simulink model "quad_tank_plant_full_sim"  (R2026a)
settings: Solver=VariableStepAuto  StopTime=120
values from neighbouring files (symbols this model uses):
  a1 = (a11 + a12)/2    [areas.m]    (also in parametros.m = 0.0006136)
  A2 = 0.159    [parametros.m]
  a2 = mean([a21 a22],2)    [areas.m]    (also in parametros.m = 0.00054678)
  A3 = 0.159    [parametros.m]
  a3 = mean([a31 a32],2)    [areas.m]    (also in parametros.m = 0.00035752; prbs_calc_L3.m = 0.00035752; ti_calc.m = 0.00035752)
  A4 = 0.159    [parametros.m]
  a4 = mean([a41 a42],2)    [areas.m]    (also in parametros.m = 0.0004182; ti_calc.m = 0.0004182)
  g = 9.81    [areas.m]    (also in parametros.m; prbs_calc_L3.m; ti_calc.m)
  gamma1 = 0.455    [areas.m]    (also in parametros.m)
  gamma2 = 0.4195    [areas.m]    (also in parametros.m)
  h_max = 0.6    [areas.m]    (also in parametros.m)
  k1 = q_max    (= 0.0017)    [areas.m]    (also in parametros.m)
  k2 = q_max    (= 0.0017)    [areas.m]    (also in parametros.m)
  q_max = 0.0017    [areas.m]    (also in parametros.m)
undefined symbols (not defined in the file or in its folder): A1
libraries: slpidlib x8, simulink x2
settings Model: Creator=agusc  LastModifiedBy=agusc

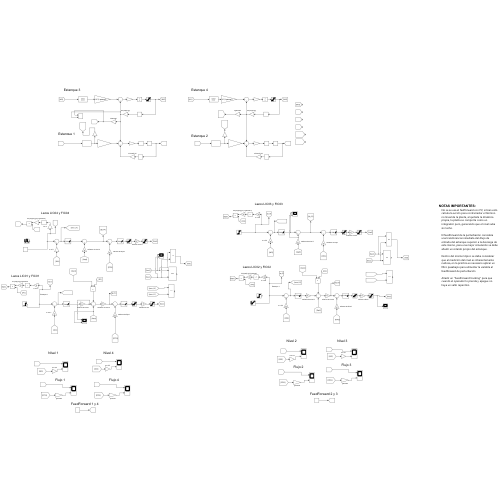
[thumbnail: Simulink's stored preview of the top-level diagram]
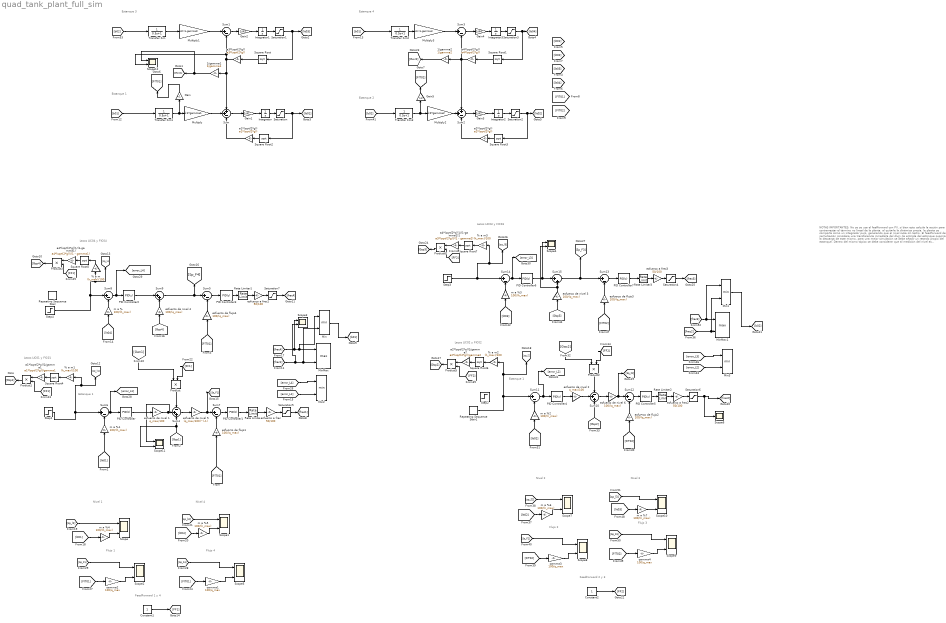
== system quad_tank_plant_full_sim ==
  note: NOTAS IMPORTANTES:
      | No se se usa el feefforward con PV, si bien esto calcula la acción para contrarrestar el término no lineal de la planta, al quitarle la dinámica propia, la planta se comporta como un integrador puro, generando que el nivel suba sin techo.
      |
      | El feedforward de la perturbación considera una transferencia inmediata del dlujo de entrada del estanque superior a la descarga de este mismo, para una mejor simulación se debe añadir un retardo propio del estanque.
      |
      | Dentro del mismo tópico se debe considerar que al medición del nivel es inherentemente ruidosa, en la práctica es necesario aplicar un filtro pasabajos para alimentar la variable al feedforward de perturbación
      |
      | Añadir un "Feedforward tracking" para que cuando el operador lo prenda y apague no haya un salto repentino
  note: Nivel 1
  note: Lazos LIC01 y FIC01
  note: Estanque 2
  note: Estanque 4
  note: Estanque 3
  note: Estanque 1
  note: Estanque 1
  note: Flujo 1
  note: Nivel 4
  note: Flujo 4
  note: FeedForward 1 y 4
  note: Lazos LIC04 y FIC04
  note: Estanque 1
  note: Lazos LIC02 y FIC02
  note: Flujo 2
  note: Nivel 2
  note: FeedForward 2 y 3
  note: Lazos LIC03 y FIC03
  note: Flujo 3
  note: Nivel 3
  % a m{,1..3} (4 alike) : Gain  Gain=(h_max)/100
  1/gamma1 : Gain  Gain=1/gamma1
  1/gamma2 : Gain  Gain=1/gamma2
  Constant1 : Constant
  Constant2 : Constant
  Gain : Gain  Gain=k1
  Gain1 : Gain  Gain=1/A1
  Gain2 : Gain  Gain=1/A3
  Gain3 : Gain  Gain=1/A2
  Gain4 : Gain  Gain=1/A4
  Gain5 : Gain  Gain=k2
  Integrator{,1..3} (4 alike) : Integrator
  Min{,1..3} (4 alike) : MinMax  Inputs=2
  MinMax : MinMax  Function=max  Inputs=2
  MinMax1 : MinMax  Function=max  Inputs=2
  Multiply : Gain  Gain=k1*gamma1
  Multiply1 : Gain  Gain=k2*(1-gamma2)
  Multiply2 : Gain  Gain=k2*gamma2
  Multiply3 : Gain  Gain=k1*(1-gamma1)
  PID Controller : slpidlib/PID Controller  Controller=PID  Form=Ideal  TimeDomain=Discrete-time  UseExternalTs=off  SampleTime=0.1  IntegratorMethod=Forward Euler  FilterMethod=Forward Euler  ControllerParametersSource=internal  P=1.125  I=0  UseKiTs=off  D=0  UseExternalDerivativeSource=off  N=100  UseFilter=on  TunerSelectOption=Transfer Function Based (PID Tuner App)  InitialConditionSource=internal  InitialConditionForIntegrator=0  InitialConditionForFilter=0  DifferentiatorICPrevScaledInput=0  ExternalReset=none  TrackingMode=off  Kt=1  LimitOutput=on  SatLimitsSource=internal  UpperSaturationLimit=100  LowerSaturationLimit=-100  LinearizeAsGain=on  AntiWindupMode=clamping  Kb=1  LimitIntegrator=off  UpperIntegratorSaturationLimit=inf  LowerIntegratorSaturationLimit=-inf  POutMin=[]  POutMax=[]  IOutMin=[]  IOutMax=[]  DOutMin=[]  DOutMax=[]  NOutMin=[]  NOutMax=[]  SumOutMin=[]  SumOutMax=[]  SaturationOutMin=[]  SaturationOutMax=[]  PParamMin=[]  PParamMax=[]  IParamMin=[]  IParamMax=[]  DParamMin=[]  DParamMax=[]  NParamMin=[]  NParamMax=[]  KbParamMin=[]  KbParamMax=[]  KtParamMin=[]  KtParamMax=[]  KbOutMin=[]  KbOutMax=[]  KtOutMin=[]  KtOutMax=[]  IntegratorOutMin=[]  IntegratorOutMax=[]  FilterOutMin=[]  FilterOutMax=[]  SumI1OutMin=[]  SumI1OutMax=[]  SumI2OutMin=[]  SumI2OutMax=[]  SumI3OutMin=[]  SumI3OutMax=[]  SumI4OutMin=[]  SumI4OutMax=[]  SumDOutMin=[]  SumDOutMax=[]  DifferentiatorOutMin=[]  DifferentiatorOutMax=[]  FilterDiffOutCoefMin=[]  FilterDiffOutCoefMax=[]  ReciprocalOutMin=[]  ReciprocalOutMax=[]  SumDenOutMin=[]  SumDenOutMax=[]  SumNumOutMin=[]  SumNumOutMax=[]  DivideOutMin=[]  DivideOutMax=[]  UdiffTsProdOutMin=[]  UdiffTsProdOutMax=[]  NTsProdOutMin=[]  NTsProdOutMax=[]  UintegralTsProdOutMin=[]  UintegralTsProdOutMax=[]  UngainTsProdOutMin=[]  UngainTsProdOutMax=[]  ClampingZeroOutDataTypeStr=Inherit: Inherit via back propagation  ClampingZeroOutMin=[]  ClampingZeroOutMax=[]  FilterDenConstantOutDataTypeStr=Inherit: Inherit via back propagation  FilterDenConstantOutMin=[]  FilterDenConstantOutMax=[]  PCopyOutDataTypeStr=Inherit: Inherit via back propagation  PCopyOutMin=[]  PCopyOutMax=[]  NCopyOutDataTypeStr=Inherit: Inherit via back propagation  NCopyOutMin=[]  NCopyOutMax=[]  IntegratorContinuousStateAttributes=''  IntegratorStateMustResolveToSignalObject=off  IntegratorRTWStateStorageClass=Auto  FilterContinuousStateAttributes=''  FilterStateMustResolveToSignalObject=off  FilterRTWStateStorageClass=Auto  ParallelPVariant=Passthrough  IdealPVariant=InternalParameters  IVariant=InternalParameters  DVariant=InternalParameters  IntegratorVariant=Discrete  SatVariant=Enabled  AWVariant=DiscClampingIdeal  PCopyVariant=InternalParamsIdeal  TRVariant=Disabled  FdbkBlocksVariant=Forward  IdealPFdbkVariant=Disabled  SatFdbkVariant=Disabled  DerivativeFilterVariant=ForwardEulerFilter  NVariant=InternalParameters  NCopyVariant=Disabled  FilterICVariant=InternalICsFilter  IntegratorICVariant=InternalICs  ExternalResetVariant=Disabled  TRSumVariant=Passthrough  SumFdbkVariant=Disabled  SumVariant=Sum_PID  TsampFilterVariant=InternalTs  TsampNgainVariant=Passthrough  TsampIntegralVariant=Disabled_SignalSpec  ExternalSaturationOutDataTypeStr=Inherit: Same as second input  DerivativeSourceVariant=ErrorSignal  PreIntVariant=InternalPreInt
  PID Controller{1,3,5,7} (4 alike) : slpidlib/PID Controller  Controller=PID  Form=Ideal  TimeDomain=Discrete-time  UseExternalTs=off  SampleTime=0.1  IntegratorMethod=Forward Euler  FilterMethod=Forward Euler  ControllerParametersSource=internal  P=1.2  I=0.485  UseKiTs=off  D=0  UseExternalDerivativeSource=off  N=100  UseFilter=on  TunerSelectOption=Transfer Function Based (PID Tuner App)  InitialConditionSource=internal  InitialConditionForIntegrator=0  InitialConditionForFilter=0  DifferentiatorICPrevScaledInput=0  ExternalReset=none  TrackingMode=off  Kt=1  LimitOutput=on  SatLimitsSource=internal  UpperSaturationLimit=100  LowerSaturationLimit=0  LinearizeAsGain=on  AntiWindupMode=none  Kb=1  LimitIntegrator=off  UpperIntegratorSaturationLimit=inf  LowerIntegratorSaturationLimit=-inf  POutMin=[]  POutMax=[]  IOutMin=[]  IOutMax=[]  DOutMin=[]  DOutMax=[]  NOutMin=[]  NOutMax=[]  SumOutMin=[]  SumOutMax=[]  SaturationOutMin=[]  SaturationOutMax=[]  PParamMin=[]  PParamMax=[]  IParamMin=[]  IParamMax=[]  DParamMin=[]  DParamMax=[]  NParamMin=[]  NParamMax=[]  KbParamMin=[]  KbParamMax=[]  KtParamMin=[]  KtParamMax=[]  KbOutMin=[]  KbOutMax=[]  KtOutMin=[]  KtOutMax=[]  IntegratorOutMin=[]  IntegratorOutMax=[]  FilterOutMin=[]  FilterOutMax=[]  SumI1OutMin=[]  SumI1OutMax=[]  SumI2OutMin=[]  SumI2OutMax=[]  SumI3OutMin=[]  SumI3OutMax=[]  SumI4OutMin=[]  SumI4OutMax=[]  SumDOutMin=[]  SumDOutMax=[]  DifferentiatorOutMin=[]  DifferentiatorOutMax=[]  FilterDiffOutCoefMin=[]  FilterDiffOutCoefMax=[]  ReciprocalOutMin=[]  ReciprocalOutMax=[]  SumDenOutMin=[]  SumDenOutMax=[]  SumNumOutMin=[]  SumNumOutMax=[]  DivideOutMin=[]  DivideOutMax=[]  UdiffTsProdOutMin=[]  UdiffTsProdOutMax=[]  NTsProdOutMin=[]  NTsProdOutMax=[]  UintegralTsProdOutMin=[]  UintegralTsProdOutMax=[]  UngainTsProdOutMin=[]  UngainTsProdOutMax=[]  ClampingZeroOutDataTypeStr=Inherit: Inherit via back propagation  ClampingZeroOutMin=[]  ClampingZeroOutMax=[]  FilterDenConstantOutDataTypeStr=Inherit: Inherit via back propagation  FilterDenConstantOutMin=[]  FilterDenConstantOutMax=[]  PCopyOutDataTypeStr=Inherit: Inherit via back propagation  PCopyOutMin=[]  PCopyOutMax=[]  NCopyOutDataTypeStr=Inherit: Inherit via back propagation  NCopyOutMin=[]  NCopyOutMax=[]  IntegratorContinuousStateAttributes=''  IntegratorStateMustResolveToSignalObject=off  IntegratorRTWStateStorageClass=Auto  FilterContinuousStateAttributes=''  FilterStateMustResolveToSignalObject=off  FilterRTWStateStorageClass=Auto  ParallelPVariant=Passthrough  IdealPVariant=InternalParameters  IVariant=InternalParameters  DVariant=InternalParameters  IntegratorVariant=Discrete  SatVariant=Enabled  AWVariant=Passthrough  PCopyVariant=Disabled  TRVariant=Disabled  FdbkBlocksVariant=Forward  IdealPFdbkVariant=Disabled  SatFdbkVariant=Disabled  DerivativeFilterVariant=ForwardEulerFilter  NVariant=InternalParameters  NCopyVariant=Disabled  FilterICVariant=InternalICsFilter  IntegratorICVariant=InternalICs  ExternalResetVariant=Disabled  TRSumVariant=Passthrough  SumFdbkVariant=Disabled  SumVariant=Sum_PID  TsampFilterVariant=InternalTs  TsampNgainVariant=Passthrough  TsampIntegralVariant=Disabled_SignalSpec  ExternalSaturationOutDataTypeStr=Inherit: Same as second input  DerivativeSourceVariant=ErrorSignal  PreIntVariant=InternalPreInt
  PID Controller2 : slpidlib/PID Controller  Controller=PID  Form=Ideal  TimeDomain=Discrete-time  UseExternalTs=off  SampleTime=0.1  IntegratorMethod=Forward Euler  FilterMethod=Forward Euler  ControllerParametersSource=internal  P=1.255  I=0  UseKiTs=off  D=0  UseExternalDerivativeSource=off  N=100  UseFilter=on  TunerSelectOption=Transfer Function Based (PID Tuner App)  InitialConditionSource=internal  InitialConditionForIntegrator=0  InitialConditionForFilter=0  DifferentiatorICPrevScaledInput=0  ExternalReset=none  TrackingMode=off  Kt=1  LimitOutput=on  SatLimitsSource=internal  UpperSaturationLimit=100  LowerSaturationLimit=0  LinearizeAsGain=on  AntiWindupMode=none  Kb=1  LimitIntegrator=off  UpperIntegratorSaturationLimit=inf  LowerIntegratorSaturationLimit=-inf  POutMin=[]  POutMax=[]  IOutMin=[]  IOutMax=[]  DOutMin=[]  DOutMax=[]  NOutMin=[]  NOutMax=[]  SumOutMin=[]  SumOutMax=[]  SaturationOutMin=[]  SaturationOutMax=[]  PParamMin=[]  PParamMax=[]  IParamMin=[]  IParamMax=[]  DParamMin=[]  DParamMax=[]  NParamMin=[]  NParamMax=[]  KbParamMin=[]  KbParamMax=[]  KtParamMin=[]  KtParamMax=[]  KbOutMin=[]  KbOutMax=[]  KtOutMin=[]  KtOutMax=[]  IntegratorOutMin=[]  IntegratorOutMax=[]  FilterOutMin=[]  FilterOutMax=[]  SumI1OutMin=[]  SumI1OutMax=[]  SumI2OutMin=[]  SumI2OutMax=[]  SumI3OutMin=[]  SumI3OutMax=[]  SumI4OutMin=[]  SumI4OutMax=[]  SumDOutMin=[]  SumDOutMax=[]  DifferentiatorOutMin=[]  DifferentiatorOutMax=[]  FilterDiffOutCoefMin=[]  FilterDiffOutCoefMax=[]  ReciprocalOutMin=[]  ReciprocalOutMax=[]  SumDenOutMin=[]  SumDenOutMax=[]  SumNumOutMin=[]  SumNumOutMax=[]  DivideOutMin=[]  DivideOutMax=[]  UdiffTsProdOutMin=[]  UdiffTsProdOutMax=[]  NTsProdOutMin=[]  NTsProdOutMax=[]  UintegralTsProdOutMin=[]  UintegralTsProdOutMax=[]  UngainTsProdOutMin=[]  UngainTsProdOutMax=[]  ClampingZeroOutDataTypeStr=Inherit: Inherit via back propagation  ClampingZeroOutMin=[]  ClampingZeroOutMax=[]  FilterDenConstantOutDataTypeStr=Inherit: Inherit via back propagation  FilterDenConstantOutMin=[]  FilterDenConstantOutMax=[]  PCopyOutDataTypeStr=Inherit: Inherit via back propagation  PCopyOutMin=[]  PCopyOutMax=[]  NCopyOutDataTypeStr=Inherit: Inherit via back propagation  NCopyOutMin=[]  NCopyOutMax=[]  IntegratorContinuousStateAttributes=''  IntegratorStateMustResolveToSignalObject=off  IntegratorRTWStateStorageClass=Auto  FilterContinuousStateAttributes=''  FilterStateMustResolveToSignalObject=off  FilterRTWStateStorageClass=Auto  ParallelPVariant=Passthrough  IdealPVariant=InternalParameters  IVariant=InternalParameters  DVariant=InternalParameters  IntegratorVariant=Discrete  SatVariant=Enabled  AWVariant=Passthrough  PCopyVariant=Disabled  TRVariant=Disabled  FdbkBlocksVariant=Forward  IdealPFdbkVariant=Disabled  SatFdbkVariant=Disabled  DerivativeFilterVariant=ForwardEulerFilter  NVariant=InternalParameters  NCopyVariant=Disabled  FilterICVariant=InternalICsFilter  IntegratorICVariant=InternalICs  ExternalResetVariant=Disabled  TRSumVariant=Passthrough  SumFdbkVariant=Disabled  SumVariant=Sum_PID  TsampFilterVariant=InternalTs  TsampNgainVariant=Passthrough  TsampIntegralVariant=Disabled_SignalSpec  ExternalSaturationOutDataTypeStr=Inherit: Same as second input  DerivativeSourceVariant=ErrorSignal  PreIntVariant=InternalPreInt
  PID Controller4 : slpidlib/PID Controller  Controller=PID  Form=Ideal  TimeDomain=Discrete-time  UseExternalTs=off  SampleTime=0.1  IntegratorMethod=Forward Euler  FilterMethod=Forward Euler  ControllerParametersSource=internal  P=1.125  I=0  UseKiTs=off  D=0  UseExternalDerivativeSource=off  N=100  UseFilter=on  TunerSelectOption=Transfer Function Based (PID Tuner App)  InitialConditionSource=internal  InitialConditionForIntegrator=0  InitialConditionForFilter=0  DifferentiatorICPrevScaledInput=0  ExternalReset=none  TrackingMode=off  Kt=1  LimitOutput=on  SatLimitsSource=internal  UpperSaturationLimit=100  LowerSaturationLimit=-100  LinearizeAsGain=on  AntiWindupMode=clamping  Kb=1  LimitIntegrator=off  UpperIntegratorSaturationLimit=inf  LowerIntegratorSaturationLimit=-inf  POutMin=[]  POutMax=[]  IOutMin=[]  IOutMax=[]  DOutMin=[]  DOutMax=[]  NOutMin=[]  NOutMax=[]  SumOutMin=[]  SumOutMax=[]  SaturationOutMin=[]  SaturationOutMax=[]  PParamMin=[]  PParamMax=[]  IParamMin=[]  IParamMax=[]  DParamMin=[]  DParamMax=[]  NParamMin=[]  NParamMax=[]  KbParamMin=[]  KbParamMax=[]  KtParamMin=[]  KtParamMax=[]  KbOutMin=[]  KbOutMax=[]  KtOutMin=[]  KtOutMax=[]  IntegratorOutMin=[]  IntegratorOutMax=[]  FilterOutMin=[]  FilterOutMax=[]  SumI1OutMin=[]  SumI1OutMax=[]  SumI2OutMin=[]  SumI2OutMax=[]  SumI3OutMin=[]  SumI3OutMax=[]  SumI4OutMin=[]  SumI4OutMax=[]  SumDOutMin=[]  SumDOutMax=[]  DifferentiatorOutMin=[]  DifferentiatorOutMax=[]  FilterDiffOutCoefMin=[]  FilterDiffOutCoefMax=[]  ReciprocalOutMin=[]  ReciprocalOutMax=[]  SumDenOutMin=[]  SumDenOutMax=[]  SumNumOutMin=[]  SumNumOutMax=[]  DivideOutMin=[]  DivideOutMax=[]  UdiffTsProdOutMin=[]  UdiffTsProdOutMax=[]  NTsProdOutMin=[]  NTsProdOutMax=[]  UintegralTsProdOutMin=[]  UintegralTsProdOutMax=[]  UngainTsProdOutMin=[]  UngainTsProdOutMax=[]  ClampingZeroOutDataTypeStr=Inherit: Inherit via back propagation  ClampingZeroOutMin=[]  ClampingZeroOutMax=[]  FilterDenConstantOutDataTypeStr=Inherit: Inherit via back propagation  FilterDenConstantOutMin=[]  FilterDenConstantOutMax=[]  PCopyOutDataTypeStr=Inherit: Inherit via back propagation  PCopyOutMin=[]  PCopyOutMax=[]  NCopyOutDataTypeStr=Inherit: Inherit via back propagation  NCopyOutMin=[]  NCopyOutMax=[]  IntegratorContinuousStateAttributes=''  IntegratorStateMustResolveToSignalObject=off  IntegratorRTWStateStorageClass=Auto  FilterContinuousStateAttributes=''  FilterStateMustResolveToSignalObject=off  FilterRTWStateStorageClass=Auto  ParallelPVariant=Passthrough  IdealPVariant=InternalParameters  IVariant=InternalParameters  DVariant=InternalParameters  IntegratorVariant=Discrete  SatVariant=Enabled  AWVariant=DiscClampingIdeal  PCopyVariant=InternalParamsIdeal  TRVariant=Disabled  FdbkBlocksVariant=Forward  IdealPFdbkVariant=Disabled  SatFdbkVariant=Disabled  DerivativeFilterVariant=ForwardEulerFilter  NVariant=InternalParameters  NCopyVariant=Disabled  FilterICVariant=InternalICsFilter  IntegratorICVariant=InternalICs  ExternalResetVariant=Disabled  TRSumVariant=Passthrough  SumFdbkVariant=Disabled  SumVariant=Sum_PID  TsampFilterVariant=InternalTs  TsampNgainVariant=Passthrough  TsampIntegralVariant=Disabled_SignalSpec  ExternalSaturationOutDataTypeStr=Inherit: Same as second input  DerivativeSourceVariant=ErrorSignal  PreIntVariant=InternalPreInt
  PID Controller6 : slpidlib/PID Controller  Controller=PID  Form=Ideal  TimeDomain=Discrete-time  UseExternalTs=off  SampleTime=0.1  IntegratorMethod=Forward Euler  FilterMethod=Forward Euler  ControllerParametersSource=internal  P=1.255  I=0  UseKiTs=off  D=0  UseExternalDerivativeSource=off  N=100  UseFilter=on  TunerSelectOption=Transfer Function Based (PID Tuner App)  InitialConditionSource=internal  InitialConditionForIntegrator=0  InitialConditionForFilter=0  DifferentiatorICPrevScaledInput=0  ExternalReset=none  TrackingMode=off  Kt=1  LimitOutput=on  SatLimitsSource=internal  UpperSaturationLimit=100  LowerSaturationLimit=0  LinearizeAsGain=on  AntiWindupMode=clamping  Kb=1  LimitIntegrator=off  UpperIntegratorSaturationLimit=inf  LowerIntegratorSaturationLimit=-inf  POutMin=[]  POutMax=[]  IOutMin=[]  IOutMax=[]  DOutMin=[]  DOutMax=[]  NOutMin=[]  NOutMax=[]  SumOutMin=[]  SumOutMax=[]  SaturationOutMin=[]  SaturationOutMax=[]  PParamMin=[]  PParamMax=[]  IParamMin=[]  IParamMax=[]  DParamMin=[]  DParamMax=[]  NParamMin=[]  NParamMax=[]  KbParamMin=[]  KbParamMax=[]  KtParamMin=[]  KtParamMax=[]  KbOutMin=[]  KbOutMax=[]  KtOutMin=[]  KtOutMax=[]  IntegratorOutMin=[]  IntegratorOutMax=[]  FilterOutMin=[]  FilterOutMax=[]  SumI1OutMin=[]  SumI1OutMax=[]  SumI2OutMin=[]  SumI2OutMax=[]  SumI3OutMin=[]  SumI3OutMax=[]  SumI4OutMin=[]  SumI4OutMax=[]  SumDOutMin=[]  SumDOutMax=[]  DifferentiatorOutMin=[]  DifferentiatorOutMax=[]  FilterDiffOutCoefMin=[]  FilterDiffOutCoefMax=[]  ReciprocalOutMin=[]  ReciprocalOutMax=[]  SumDenOutMin=[]  SumDenOutMax=[]  SumNumOutMin=[]  SumNumOutMax=[]  DivideOutMin=[]  DivideOutMax=[]  UdiffTsProdOutMin=[]  UdiffTsProdOutMax=[]  NTsProdOutMin=[]  NTsProdOutMax=[]  UintegralTsProdOutMin=[]  UintegralTsProdOutMax=[]  UngainTsProdOutMin=[]  UngainTsProdOutMax=[]  ClampingZeroOutDataTypeStr=Inherit: Inherit via back propagation  ClampingZeroOutMin=[]  ClampingZeroOutMax=[]  FilterDenConstantOutDataTypeStr=Inherit: Inherit via back propagation  FilterDenConstantOutMin=[]  FilterDenConstantOutMax=[]  PCopyOutDataTypeStr=Inherit: Inherit via back propagation  PCopyOutMin=[]  PCopyOutMax=[]  NCopyOutDataTypeStr=Inherit: Inherit via back propagation  NCopyOutMin=[]  NCopyOutMax=[]  IntegratorContinuousStateAttributes=''  IntegratorStateMustResolveToSignalObject=off  IntegratorRTWStateStorageClass=Auto  FilterContinuousStateAttributes=''  FilterStateMustResolveToSignalObject=off  FilterRTWStateStorageClass=Auto  ParallelPVariant=Passthrough  IdealPVariant=InternalParameters  IVariant=InternalParameters  DVariant=InternalParameters  IntegratorVariant=Discrete  SatVariant=Enabled  AWVariant=DiscClampingIdeal  PCopyVariant=InternalParamsIdeal  TRVariant=Disabled  FdbkBlocksVariant=Forward  IdealPFdbkVariant=Disabled  SatFdbkVariant=Disabled  DerivativeFilterVariant=ForwardEulerFilter  NVariant=InternalParameters  NCopyVariant=Disabled  FilterICVariant=InternalICsFilter  IntegratorICVariant=InternalICs  ExternalResetVariant=Disabled  TRSumVariant=Passthrough  SumFdbkVariant=Disabled  SumVariant=Sum_PID  TsampFilterVariant=InternalTs  TsampNgainVariant=Passthrough  TsampIntegralVariant=Disabled_SignalSpec  ExternalSaturationOutDataTypeStr=Inherit: Same as second input  DerivativeSourceVariant=ErrorSignal  PreIntVariant=InternalPreInt
  Product{,1..3,5..6} (6 alike) : Product
  Rate Limiter{,1..3} (4 alike) : RateLimiter  RisingSlewLimit=20  FallingSlewLimit=-20  SampleTimeMode=inherited
  Repeating Sequence Stair : simulink/Sources/Repeating Sequence Stair  OutValues=[20 70 20].'  tsamp=40  OutMin=[]  OutMax=[]  OutDataTypeStr=double  OutputDataTypeScalingMode=double  OutDataType=fixdt(0,8)  ConRadixGroup=Best Precision: Vector-wise  OutScaling=2^-12
  Repeating Sequence Stair1 : simulink/Sources/Repeating Sequence Stair  OutValues=[30 50 70].'  tsamp=40  OutMin=[]  OutMax=[]  OutDataTypeStr=double  OutputDataTypeScalingMode=double  OutDataType=fixdt(0,8)  ConRadixGroup=Best Precision: Vector-wise  OutScaling=2^-12
  Saturation{,1..3} (4 alike) : Saturate  UpperLimit=h_max  LowerLimit=0
  Saturation{4..7} (4 alike) : Saturate  UpperLimit=50  LowerLimit=0
  Scope{,1..5,7..10,12} (11 alike) : Scope  NumInputPorts=2
      Scope settings: ActiveDisplayYMinimum=-12.499999999999996  ActiveDisplayYMaximum=112.5
      Scope1 settings: ActiveDisplayYMinimum=-8.2680207313095071  ActiveDisplayYMaximum=74.412186581785576
      Scope10 settings: ActiveDisplayYMinimum=-6.2499999999999982  ActiveDisplayYMaximum=56.25  DataLoggingVariableName=ScopeData10
      Scope12 settings: ActiveDisplayYMinimum=-0.00043820457402529234  ActiveDisplayYMaximum=0.0022511243567603493  DataLoggingVariableName=ScopeData12
      Scope2 settings: ActiveDisplayYMinimum=-18.95496582345929  ActiveDisplayYMaximum=132.60230226797611  DataLoggingVariableName=ScopeData2
      Scope3 settings: ActiveDisplayYMinimum=-6.2499999999999982  ActiveDisplayYMaximum=56.25  DataLoggingVariableName=ScopeData3
      Scope4 settings: ActiveDisplayYMinimum=-100.91570319464546  ActiveDisplayYMaximum=108.60777038049341  DataLoggingVariableName=ScopeData4
      Scope5 settings: ActiveDisplayYMinimum=-15.074553877755356  ActiveDisplayYMaximum=61.05405346388288  DataLoggingVariableName=ScopeData5
      Scope7 settings: ActiveDisplayYMinimum=-12.499999999999996  ActiveDisplayYMaximum=112.5  DataLoggingVariableName=ScopeData7
      Scope8 settings: ActiveDisplayYMinimum=-72.129298571446512  ActiveDisplayYMaximum=111.88845498606268  DataLoggingVariableName=ScopeData8
      Scope9 settings: ActiveDisplayYMinimum=-6.2568668761095019  ActiveDisplayYMaximum=56.374326786315692  DataLoggingVariableName=ScopeData9
  Scope11 : Scope  NumInputPorts=3
      settings: ActiveDisplayYMinimum=-0.0003749999999999999  ActiveDisplayYMaximum=0.003375  DataLoggingVariableName=ScopeData11
  Scope6 : Scope
      settings: ActiveDisplayYMinimum=-10.918861993908987  ActiveDisplayYMaximum=98.2697579451809  DataLoggingVariableName=ScopeData6
  Square Root{,1..7} (8 alike) : Sqrt
  Step1 : Step  InitialValue=10  FinalValue=50  SampleTime=0
  Step2 : Step  FinalValue=50  SampleTime=0
  Step3 : Step  FinalValue=50  SampleTime=0
  Step4 : Step  FinalValue=50  SampleTime=0
  Sum : Sum  Inputs=++-
  Sum{1,3,5..8,11..14} (10 alike) : Sum  Inputs=|+-
  Sum10 : Sum  Inputs=-++
  Sum15 : Sum  Inputs=|++
  Sum2 : Sum  Inputs=++-
  Sum4 : Sum  Inputs=-++
  Sum9 : Sum  Inputs=|++
  Transfer Fcn{,1..3} (4 alike) : TransferFcn  Denominator=[0.5 1]
  a1*(sqrt(2*g)) : Gain  Gain=a1*(sqrt(2*g))
  a1*(sqrt(2*g))1/gamma1 : Gain  Gain=a1*(sqrt(2*g))/gamma1
  a2*(sqrt(2*g)) : Gain  Gain=a2*(sqrt(2*g))
  a2*(sqrt(2*g))1/gamma2 : Gain  Gain=a2*(sqrt(2*g))/gamma2
  a3*(sqrt(2*g)) : Gain  Gain=a3*(sqrt(2*g))
  a4*(sqrt(2*g)) : Gain  Gain=a4*(sqrt(2*g))
  a4*(sqrt(2*g))1/(1-gamma1) : Gain  Gain=a4*(sqrt(2*g))/(1 - gamma1)
  a4*(sqrt(2*g))1/(1-gamma1)1 : Gain  Gain=a3*(sqrt(2*g))/(1 - gamma2)
  esfuerzo a frec{,1..3} (4 alike) : Gain  Gain=50/100
  esfuerzo de flujo{1..4} (4 alike) : Gain  Gain=100/(q_max)
  esfuerzo de nivel 1 : Gain  Gain=q_max/100
  esfuerzo de nivel 2 : Gain  Gain=q_max/100
  esfuerzo de nivel 3 : Gain  Gain=100/(q_max)
  esfuerzo de nivel 4 : Gain  Gain=100/(q_max)
  esfuerzo de nivel 5 : Gain  Gain=(q_max/100)^(-1)
  esfuerzo de nivel 6 : Gain  Gain=100/(q_max)
  gamma{1..4} (4 alike) : Gain  Gain=100/q_max
  m a %{,1..7} (8 alike) : Gain  Gain=100/(h_max)
  wires:
  Square Root/1 -> a3*(sqrt(2*g))/1
  a1*(sqrt(2*g))/1 -> Sum/3
  Square Root2/1 -> a1*(sqrt(2*g))/1
  Saturation1/1 -> [lit03], Square Root/1
  Multiply1/1 -> Sum1/1
  a3*(sqrt(2*g))/1 -> Scope12/2, Sum1/2, Sum/1, 1/gamma1/1
  Saturation/1 -> [lit01], Square Root2/1
  Gain1/1 -> Integrator/1
  Multiply3/1 -> Sum3/1
  Saturation2/1 -> [lit02], Square Root3/1
  a4*(sqrt(2*g))/1 -> 1/gamma2/1, Sum2/1, Sum3/2
  Multiply2/1 -> Sum2/2
  a2*(sqrt(2*g))/1 -> Sum2/3
  Square Root1/1 -> a4*(sqrt(2*g))/1
  Sum2/1 -> Gain3/1
  Gain4/1 -> Integrator3/1
  Saturation3/1 -> [lit04], Square Root1/1
  Square Root3/1 -> a2*(sqrt(2*g))/1
  Sum1/1 -> Gain2/1
  Gain2/1 -> Integrator1/1
  Integrator1/1 -> Saturation1/1
  Sum/1 -> Gain1/1
  Integrator/1 -> Saturation/1
  Integrator2/1 -> Saturation2/1
  Gain3/1 -> Integrator2/1
  Sum3/1 -> Gain4/1
  Integrator3/1 -> Saturation3/1
  Transfer Fcn/1 -> Multiply1/1
  [b01] -> Transfer Fcn1/1
  Transfer Fcn1/1 -> Gain/1, Multiply/1
  Transfer Fcn2/1 -> Multiply3/1
  Gain/1 -> [FIT01]
  Transfer Fcn3/1 -> Gain5/1, Multiply2/1
  Gain5/1 -> [FIT02]
  Sum6/1 -> [error_L1], PID Controller/1
  Sum7/1 -> PID Controller1/1
  [Gsp1] -> Scope11/3, Sum4/3
  Square Root4/1 -> a1*(sqrt(2*g))1/gamma1/1
  a1*(sqrt(2*g))1/gamma1/1 -> Product1/1
  [lit04] -> m a %/1
  Sum8/1 -> [error_L4], PID Controller2/1
  a4*(sqrt(2*g))1/(1-gamma1)/1 -> Product3/1
  Step1/1 -> Sum6/1, % a m1/1, [sp_l1]
  Square Root5/1 -> a4*(sqrt(2*g))1/(1-gamma1)/1
  PID Controller3/1 -> Rate Limiter1/1
  [lit01] -> m a %4/1
  [sp_l1] -> Scope/1
  [lit04] -> m a %5/1
  [sp_l4] -> Scope1/1
  [FF1] -> Product/2
  Product/1 -> Sum4/1
  Product1/1 -> [Gsp1]
  [FF1] -> Product1/2
  Product3/1 -> [Gsp4]
  [FF1] -> Product3/2
  [FIT01] -> gamma2/1
  [Sp_F1] -> Scope2/1
  Multiply/1 -> Sum/2
  gamma2/1 -> Scope2/2
  esfuerzo a frec/1 -> Saturation5/1
  [FIT01] -> esfuerzo de flujo1/1
  esfuerzo de flujo1/1 -> Sum7/2
  Rate Limiter/1 -> esfuerzo a frec/1
  Sum5/1 -> PID Controller3/1
  esfuerzo de flujo4/1 -> Sum5/2
  [FIT01] -> esfuerzo de flujo4/1
  [Sp_F4] -> Scope5/1
  [FIT01] -> gamma1/1
  gamma1/1 -> Scope5/2
  Rate Limiter1/1 -> esfuerzo a frec1/1
  esfuerzo a frec1/1 -> Saturation7/1
  [FIT02] -> esfuerzo de flujo2/1
  Rate Limiter2/1 -> esfuerzo a frec2/1
  esfuerzo a frec2/1 -> Saturation6/1
  Repeating Sequence Stair1/1 -> % a m2/1, [sp_l2], Sum11/1
  a2*(sqrt(2*g))1/gamma2/1 -> Product5/1
  Sum11/1 -> [error_L2], PID Controller4/1
  Sum12/1 -> PID Controller5/1
  Product2/1 -> Sum10/1
  Product5/1 -> [Gsp2]
  PID Controller4/1 -> esfuerzo de nivel 2/1
  esfuerzo de flujo2/1 -> Sum12/2
  [Gsp2] -> Sum10/3
  [FF2] -> Product5/2
  [lit02] -> m a %2/1
  PID Controller5/1 -> Rate Limiter2/1
  [FF2] -> Product2/2
  Square Root6/1 -> a2*(sqrt(2*g))1/gamma2/1
  [Sp_F2] -> Scope8/1
  [sp_l2] -> Scope7/1
  [FIT02] -> gamma3/1
  [lit02] -> m a %6/1
  gamma3/1 -> Scope8/2
  Constant2/1 -> [FF2]
  1/gamma2/1 -> [Gwc2]
  [b02] -> Transfer Fcn3/1
  [FIT02] -> esfuerzo de flujo3/1
  Sum13/1 -> PID Controller7/1
  esfuerzo a frec3/1 -> Saturation4/1
  [FF2] -> Product6/2
  a4*(sqrt(2*g))1/(1-gamma1)1/1 -> Product6/1
  Sum14/1 -> [error_L3], PID Controller6/1
  [Gsp3] -> esfuerzo de nivel 3/1
  PID Controller7/1 -> Rate Limiter3/1
  Rate Limiter3/1 -> esfuerzo a frec3/1
  Square Root7/1 -> a4*(sqrt(2*g))1/(1-gamma1)1/1
  esfuerzo de flujo3/1 -> Sum13/2
  PID Controller6/1 -> Scope4/1, Sum15/1
  Product6/1 -> [Gsp3]
  [lit03] -> m a %3/1
  [FIT02] -> gamma4/1
  gamma4/1 -> Scope9/2
  [Sp_F3] -> Scope9/1
  [lit03] -> m a %7/1
  [sp_l3] -> Scope10/1
  PID Controller2/1 -> Sum9/1
  [Gsp4] -> esfuerzo de nivel 4/1
  % a m/1 -> Square Root5/1
  m a %/1 -> Sum8/2
  m a %1/1 -> Sum6/2
  m a %2/1 -> Sum11/2
  % a m2/1 -> Square Root6/1
  % a m3/1 -> Square Root7/1
  m a %3/1 -> Sum14/2
  Sum15/1 -> Sum13/1, [Sp_F3]
  m a %4/1 -> Scope/2
  m a %5/1 -> Scope1/2
  esfuerzo de nivel 2/1 -> Sum10/2
  Sum10/1 -> esfuerzo de nivel 6/1
  Sum4/1 -> esfuerzo de nivel 5/1
  esfuerzo de nivel 5/1 -> [Sp_F1], Sum7/1
  PID Controller/1 -> esfuerzo de nivel 1/1
  m a %6/1 -> Scope7/2
  esfuerzo de nivel 6/1 -> [Sp_F2], Sum12/1
  [frec4] -> Min/1, MinMax/1, Scope3/1
  esfuerzo de nivel 4/1 -> Sum9/2
  Sum9/1 -> Sum5/1, [Sp_F4]
  Step3/1 -> % a m3/1, [sp_l3], Sum14/1
  [b01] -> Transfer Fcn2/1
  m a %7/1 -> Scope10/2
  Saturation4/1 -> [frec3]
  Saturation7/1 -> [frec4]
  PID Controller1/1 -> Rate Limiter/1
  Saturation5/1 -> [frec1]
  Constant1/1 -> [FF1]
  [b02] -> Transfer Fcn/1
  1/gamma1/1 -> Scope12/1, [Gwc1]
  esfuerzo de nivel 1/1 -> Scope11/1, Sum4/2
  esfuerzo de nivel 3/1 -> Scope4/2, Sum15/2
  [frec2] -> Min1/2, MinMax1/2
  Step4/1 -> % a m/1, [sp_l4], Sum8/1
  [frec1] -> Scope3/2, Min/2, MinMax/2
  [Gwc1] -> Product/1
  [Gwc2] -> Product2/1
  [lit01] -> m a %1/1
  % a m1/1 -> Square Root4/1
  [frec3] -> Min1/1, MinMax1/1
  Saturation6/1 -> Scope6/1, [frec2]
  [error_L1] -> Min2/2
  [error_L4] -> Min2/1
  [error_L2] -> Min3/2
  [error_L3] -> Min3/1
  Min/1 -> [b01]
  Min1/1 -> [b02]
